simulink subsystem "WIW2025InvSub"  (R2024b)
settings: Solver=VariableStepAuto  StartTime=0.0  StopTime=10.0  RelTol=1e-3
values from neighbouring files (symbols this model uses):
  p =     [parInvP0_0.2.mat]    (also in parInvP0_0.4.mat; parInvP0_0.6.mat; parInvP0_0.8.mat)
  parInvLinMdl =     [parInvP0_0.2.mat]    (also in parInvP0_0.4.mat; parInvP0_0.6.mat; parInvP0_0.8.mat)
settings Model: Creator=jb  LastModifiedBy=jb

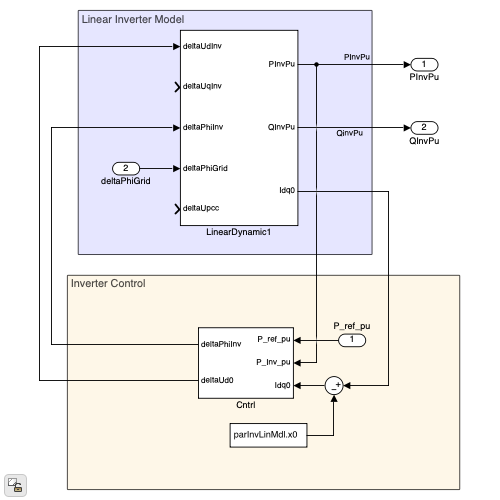
[thumbnail: Simulink's stored preview of the top-level diagram]
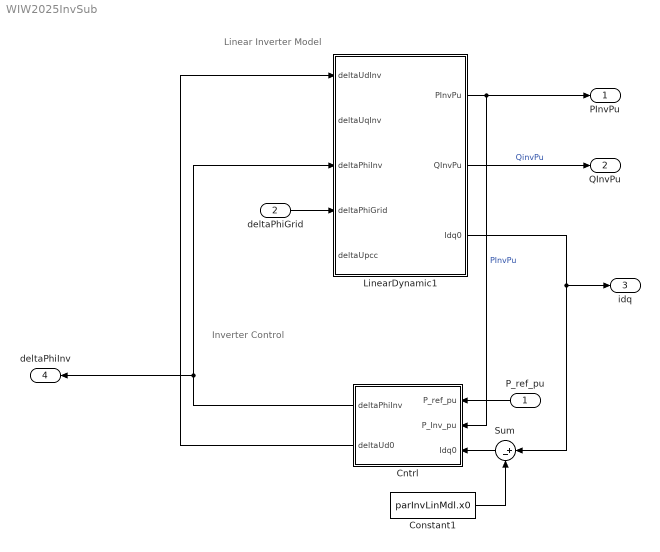
== system WIW2025InvSub ==
  note: Linear Inverter Model
  note: Inverter Control
  P_ref_pu : Inport
  deltaPhiGrid : Inport  Port=2
  Cntrl : Subsystem
  Constant1 : Constant  Value=parInvLinMdl.x0
  LinearDynamic1 : Subsystem
  Sum : Sum  Inputs=|+-
  PInvPu : Outport
  QInvPu : Outport  Port=2
  idq : Outport  Port=3
  deltaPhiInv : Outport  Port=4
  wires:
  deltaPhiGrid/1 -> LinearDynamic1/4(deltaPhiGrid)
  LinearDynamic1/3(Idq0) -> Sum/1, idq/1
  Cntrl/1(deltaPhiInv) -> LinearDynamic1/3(deltaPhiInv), deltaPhiInv/1
  Cntrl/2(deltaUd0) -> LinearDynamic1/1(deltaUdInv)
  LinearDynamic1/2(QInvPu) -> QInvPu/1  "QinvPu"
  LinearDynamic1/1(PInvPu) -> Cntrl/2(P_Inv_pu), PInvPu/1  "PInvPu"
  Sum/1 -> Cntrl/3(Idq0)
  Constant1/1 -> Sum/2
  P_ref_pu/1 -> Cntrl/1(P_ref_pu)

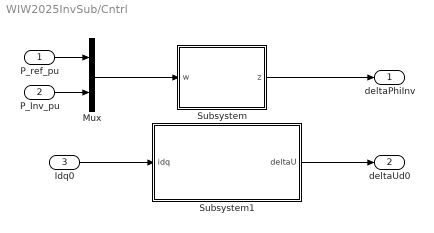
== system WIW2025InvSub/Cntrl ==
  P_ref_pu : Inport
  P_Inv_pu : Inport  Port=2
  Idq0 : Inport  Port=3
  Mux : Mux  Inputs=2
  Subsystem : Subsystem
  Subsystem1 : Subsystem
  deltaPhiInv : Outport
  deltaUd0 : Outport  Port=2
  wires:
  P_Inv_pu/1 -> Mux/2
  P_ref_pu/1 -> Mux/1
  Mux/1 -> Subsystem/1(w)
  Subsystem/1(z) -> deltaPhiInv/1
  Subsystem1/1(deltaU) -> deltaUd0/1
  Idq0/1 -> Subsystem1/1(idq)

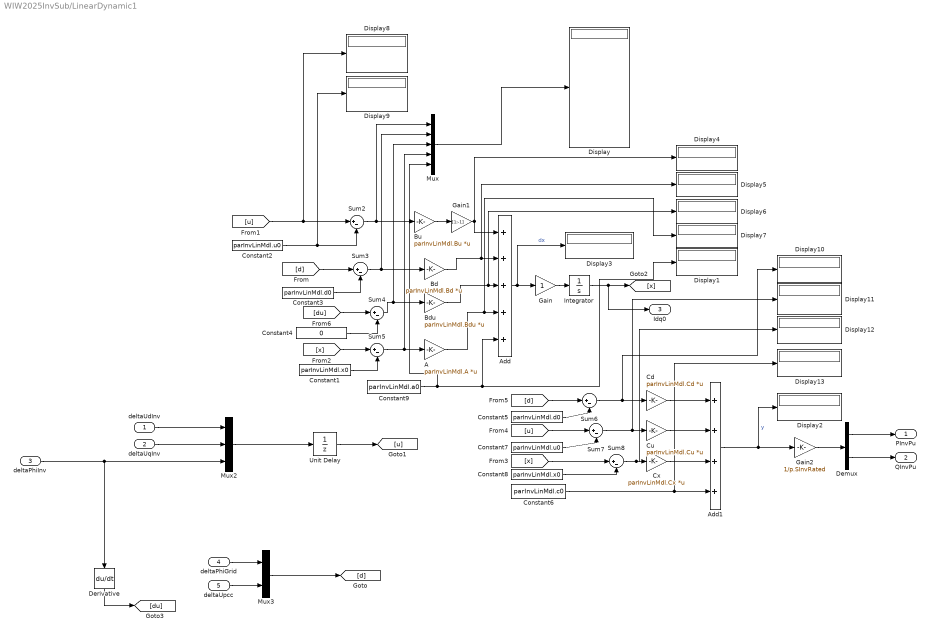
== system WIW2025InvSub/LinearDynamic1 ==
  deltaUdInv : Inport
  deltaUqInv : Inport  Port=2
  deltaPhiInv : Inport  Port=3
  deltaPhiGrid : Inport  Port=4
  deltaUpcc : Inport  Port=5
  A : Gain  Gain=parInvLinMdl.A  Multiplication=Matrix(K*u)
  Add : Sum  Inputs=+++++
  Add1 : Sum  Inputs=++++
  Bd : Gain  Gain=parInvLinMdl.Bd  Multiplication=Matrix(K*u)
  Bdu : Gain  Gain=parInvLinMdl.Bdu  Multiplication=Matrix(K*u)
  Bu : Gain  Gain=parInvLinMdl.Bu  Multiplication=Matrix(K*u)
  Cd : Gain  Gain=parInvLinMdl.Cd  Multiplication=Matrix(K*u)
  Constant1 : Constant  Value=parInvLinMdl.x0
  Constant2 : Constant  Value=parInvLinMdl.u0
  Constant3 : Constant  Value=parInvLinMdl.d0
  Constant4 : Constant  Value=0
  Constant5 : Constant  Value=parInvLinMdl.d0
  Constant6 : Constant  Value=parInvLinMdl.c0
  Constant7 : Constant  Value=parInvLinMdl.u0
  Constant8 : Constant  Value=parInvLinMdl.x0
  Constant9 : Constant  Value=parInvLinMdl.a0
  Cu : Gain  Gain=parInvLinMdl.Cu  Multiplication=Matrix(K*u)
  Cx : Gain  Gain=parInvLinMdl.Cx  Multiplication=Matrix(K*u)
  Demux : Demux  Outputs=2
  Derivative : Derivative
  Display{,1..13} (14 alike) : Display
  Gain : Gain
  Gain1 : Gain  Gain=[1;-1]
  Gain2 : Gain  Gain=1/p.SInvRated
  Integrator : Integrator  InitialCondition=parInvLinMdl.x0
  Mux : Mux  Inputs=5
  Mux2 : Mux  Inputs=3
  Mux3 : Mux  Inputs=2
  Sum{2..8} (7 alike) : Sum  Inputs=|+-
  Unit Delay : UnitDelay  SampleTime=-1  HasFrameUpgradeWarning=on
  PInvPu : Outport
  QInvPu : Outport  Port=2
  Idq0 : Outport  Port=3
  wires:
  Cu/1 -> Add1/2
  deltaUqInv/1 -> Mux2/2
  Add/1 -> Gain/1, Display3/1  "dx"
  Add1/1 -> Display2/1, Gain2/1  "y"
  Gain/1 -> Integrator/1
  Unit Delay/1 -> [u]
  deltaUpcc/1 -> Mux3/2
  Derivative/1 -> [du]
  Constant6/1 -> Add1/4, Display13/1
  Demux/1 -> PInvPu/1
  Cx/1 -> Add1/3
  Mux3/1 -> [d]
  Gain2/1 -> Demux/1
  deltaPhiInv/1 -> Derivative/1, Mux2/3
  Constant5/1 -> Sum6/2
  [du] -> Sum4/1
  Bd/1 -> Add/2, Display5/1
  Sum5/1 -> Mux/4, A/1
  [x] -> Sum5/1
  Sum7/1 -> Cu/1, Display11/1
  Sum2/1 -> Mux/1, Bu/1
  Cd/1 -> Add1/1
  Bdu/1 -> Add/3, Display6/1
  A/1 -> Display7/1, Add/4
  Constant3/1 -> Sum3/2
  [d] -> Sum6/1
  Constant9/1 -> Display1/1, Add/5, Mux/5
  Bu/1 -> Gain1/1
  deltaPhiGrid/1 -> Mux3/1
  [u] -> Sum7/1
  Sum8/1 -> Cx/1, Display12/1
  deltaUdInv/1 -> Mux2/1
  Constant7/1 -> Sum7/2
  Sum4/1 -> Mux/3, Bdu/1
  [x] -> Sum8/1
  Constant4/1 -> Sum4/2
  Mux/1 -> Display/1
  [d] -> Sum3/1
  Integrator/1 -> [x], Idq0/1
  Constant1/1 -> Sum5/2
  Constant8/1 -> Sum8/2
  [u] -> Display8/1, Sum2/1
  Demux/2 -> QInvPu/1
  Sum3/1 -> Mux/2, Bd/1
  Sum6/1 -> Cd/1, Display10/1
  Constant2/1 -> Display9/1, Sum2/2
  Mux2/1 -> Unit Delay/1
  Gain1/1 -> Add/1, Display4/1

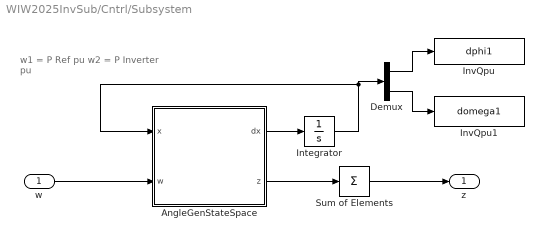
== system WIW2025InvSub/Cntrl/Subsystem ==
  note: w1 = P Ref pu
      | w2 = P Inverter pu
  w : Inport
  AngleGenStateSpace : MATLAB Function  TreatAsAtomicUnit=on
  Demux : Demux  Outputs=2
  Integrator : Integrator  InitialCondition=[0;0]
  InvQpu : ToWorkspace  VariableName=dphi1  SaveFormat=Structure With Time  SampleTime=-1
  InvQpu1 : ToWorkspace  VariableName=domega1  SaveFormat=Structure With Time  SampleTime=-1
  Sum of Elements : Sum  Inputs=+
  z : Outport
  wires:
  Demux/2 -> InvQpu1/1
  w/1 -> AngleGenStateSpace/2(w)
  AngleGenStateSpace/1(dx) -> Integrator/1
  Demux/1 -> InvQpu/1
  Integrator/1 -> AngleGenStateSpace/1(x), Demux/1
  AngleGenStateSpace/2(z) -> Sum of Elements/1
  Sum of Elements/1 -> z/1

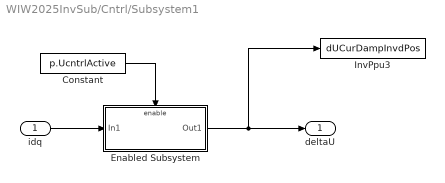
== system WIW2025InvSub/Cntrl/Subsystem1 ==
  idq : Inport  PortDimensions=2
  Constant : Constant  Value=p.UcntrlActive
  Enabled Subsystem : Subsystem  TreatAsAtomicUnit=on
  InvPpu3 : ToWorkspace  VariableName=dUCurDampInvdPos  SaveFormat=Structure With Time  SampleTime=-1
  deltaU : Outport
  wires:
  idq/1 -> Enabled Subsystem/1(In1)
  Enabled Subsystem/1(Out1) -> deltaU/1, InvPpu3/1
  Constant/1 -> Enabled Subsystem/Enable

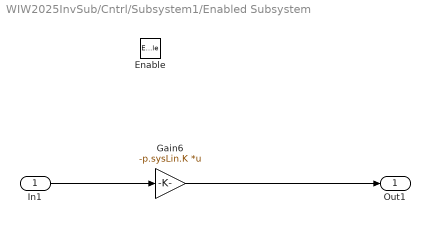
== system WIW2025InvSub/Cntrl/Subsystem1/Enabled Subsystem ==
  In1 : Inport
  Enable : EnablePort
  Gain6 : Gain  Gain=-p.sysLin.K  Multiplication=Matrix(K*u)
  Out1 : Outport
  wires:
  Gain6/1 -> Out1/1
  In1/1 -> Gain6/1

== matlab function WIW2025InvSub/Cntrl/Subsystem/AngleGenStateSpace ==
  data: x input; w input; dx output; z output; p parameter
function [dx,z]  = fcn(x,w,p)
LTIAngleGen = p.LTIAngleGen;
A = LTIAngleGen.A;
Bw = LTIAngleGen.Bw;
Cz = LTIAngleGen.Cz;
Dzw = LTIAngleGen.Dzw;


dx = A*x+Bw*w;
z = Cz*x+Dzw*w;
